simulink model "path_detector"  (Simulink 7.6)
settings: Solver=FixedStepDiscrete  StartTime=0.0  StopTime=0  RelTol=1e-3
values from neighbouring files (symbols this model uses):
  Down_Camera_Dimensions = [120 160]    [VisionConstants.m]
  Iter_Segment_Thresh = 60    [VisionConstants.m]
undefined symbols (not defined in the file or in its folder): a_range, b_range, Rec, SDTV
libraries: vipgeotforms x3, vipconversions x2, viptextngfix x2, viptransforms x2, vipanalysis x1
settings Model: Creator=auvt  LastModifiedBy=auvt  ParamWorkspaceSource=ReferencedWorkspace  TunableVars=Compass_Yaw_Kd,Compass_Yaw_Ki,Compass_Yaw_Kp,Depth_Kd,Depth_Ki,Depth_Kp,Heading_Kd,Heading_Ki,Heading_Kp,IMU_YVel_Kd,IMU_YVel_Ki,IMU_YVel_Kp,IMU_YawRate_Kd,IMU_YawRate_Ki,IMU_YawRate_Kp,Target_Down_X_Kd,Target_Down_X_Ki,Target_Down_X_Kp,Target_Down_Y_Kd,Target_Down_Y_Ki,Target_Down_Y_Kp,Target_Down_Yaw_Kd,Target_Down_Yaw_Ki,Target_Down_Yaw_Kp,Target_Forward_Y_Kd,Target_Forward_Y_Ki,Target_Forward_Y_Kp,Target_Forward_Yaw_Kd,Target_Forward_Yaw_Ki,Target_Forward_Yaw_Kp,Target_Forward_Z_Kd,Target_Forward_Z_Ki,Target_Forward_Z_Kp,Thruster_Friction_Zero,Thruster_LeftAngled_Gain,Thruster_LeftFwd_Gain,Thruster_RightAngled_Gain,Thruster_RightFwd_Gain,ZVelocity_Neg_Max  TunableVarsStorageClass=Auto,Auto,Auto,Auto,Auto,Auto,Auto,Auto,Auto,Auto,Auto,Auto,Auto,Auto,Auto,Auto,Auto,Auto,Auto,Auto,Auto,Auto,Auto,Auto,Auto,Auto,Auto,Auto,Auto,Auto,Auto,Auto,Auto,Auto,Auto,Auto,Auto,Auto,Auto  TunableVarsTypeQualifier=,,,,,,,,,,,,,,,,,,,,,,,,,,,,,,,,,,,,,,
settings MATStruct: SampleTime=0.02  Offset=0  Priority=[1.0]
settings OptimizationCC: InlineParams=on  OptimizeModelRefInitCode=on
settings RTWCC: SystemTargetFile=ert.tlc  GenCodeOnly=on  TemplateMakefile=ert_default_tmf  PostCodeGenCommand=packNGo(buildInfo);  Description=Real-Time Workshop Embedded Coder  GenerateReport=on  ProcessScript=ert_make_rtw_hook  IncludeHyperlinkInReport=on  LaunchReport=on  TargetLang=C++
settings CodeAppCC: IgnoreCustomStorageClasses=off
settings ERTTargetCC: MultiwordLength=2048  GenerateSampleERTMain=on  IncludeMdlTerminateFcn=off  InlinedParameterPlacement=NonHierarchical  ERTCustomFileTemplate=example_file_process.tlc  ConvertIfToSwitch=off

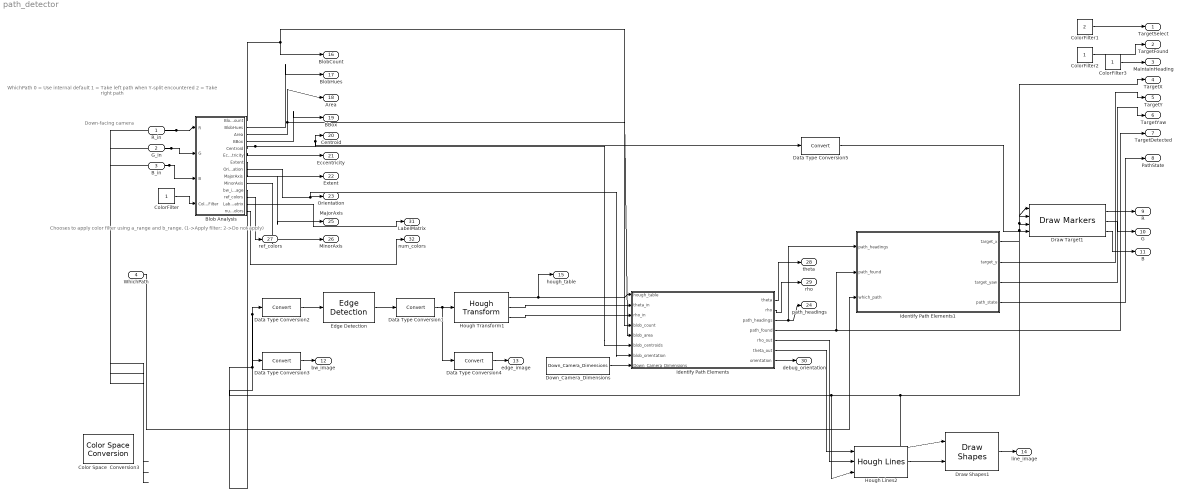
== system path_detector ==
  note: Down-facing camera
  note: WhichPath
      | 0 = Use internal default
      | 1 = Take left path when Y-split encountered
      | 2 = Take right path
  note: Chooses to apply color
      | filter using a_range and
      | b_range. (1->Apply
      | filter; 2->Do not apply)
  R_in : Inport  PortDimensions=Down_Camera_Dimensions
  G_in : Inport  Port=2  PortDimensions=Down_Camera_Dimensions
  B_in : Inport  Port=3  PortDimensions=Down_Camera_Dimensions
  WhichPath : Inport  Port=4
  Blob Analysis : Subsystem
  Color Space  Conversion3 : vipconversions/Color Space  Conversion  conversion=Obsolete  conversionActive=R'G'B' to HSV  wp_str=D50  rec=Rec. 601 (SDTV)  sys=1125/60/2:1  imagePorts=Separate color signals
  ColorFilter : Constant  SampleTime=-1
  ColorFilter1 : Constant  Value=2  SampleTime=-1
  ColorFilter2 : Constant  SampleTime=-1
  ColorFilter3 : Constant  SampleTime=-1
  Data Type Conversion{1..5} (5 alike) : DataTypeConversion
  Down_Camera_Dimensions : Constant  Value=Down_Camera_Dimensions  SampleTime=-1
  Draw Shapes1 : viptextngfix/Draw Shapes  DialogController=vipDDGCreate  DialogControllerArgs=DataTag3  shape=Lines  fill=off  fillClrSource=Specify via dialog  display=User-specified value  intensity=200  color=.2  opacity=0.6  viewport=Entire image  antialiasing=off  inType=Obsolete  imagePorts=One multidimensional signal  prodOutputMode=Binary point scaling  prodOutputWordLength=32  prodOutputFracLength=14  memoryMode=Specify word length  memoryWordLength=16  memoryFracLength=15  roundingMode=Floor  overflowMode=off
  Draw Target1 : viptextngfix/Draw Markers  DialogController=vipDDGCreate  DialogControllerArgs=DataTag4  shape=X-mark  size=7  fill=off  fillClrSource=Specify via dialog  display=Black  intensity=200  color=[0 0 0]  opacity=0.6  viewport=Entire image  antialiasing=off  inType=Obsolete  imagePorts=Separate color signals  prodOutputMode=Binary point scaling  prodOutputWordLength=32  prodOutputFracLength=14  memoryMode=Specify word length  memoryWordLength=16  memoryFracLength=15  roundingMode=Floor  overflowMode=off
  Edge Detection : vipanalysis/Edge Detection  DialogController=vipDDGCreate  DialogControllerArgs=DataTag5  method=Sobel  outputType=Binary image  userDefinedThreshold=off  thresholdSource=Specify via dialog  threshold=20  thresholdTuning=3  edgeThinning=on  threshold_canny=[0.25 0.60]  autoPercent=70  sigma=1  roundingMode=Floor  overflowMode=off
  Hough Lines2 : viptransforms/Hough Lines  DialogController=vipDDGCreate  DialogControllerArgs=DataTag6  sineCompMethod=Trigonometric function  thetaRes=pi/180  firstCoeffMode=Specify word length  firstCoeffWordLength=16  firstCoeffFracLength=15  prodOutputMode=Binary point scaling  prodOutputWordLength=32  prodOutputFracLength=16  roundingMode=Nearest  overflowMode=on
  Hough Transform1 : viptransforms/Hough Transform  DialogController=vipDDGCreate  DialogControllerArgs=DataTag7  theta_res=pi/180  rho_res=1  out_theta_rho=on  outdtmode=double  firstCoeffMode=Binary point scaling  firstCoeffWordLength=16  firstCoeffFracLength=14  secondCoeffMode=Binary point scaling  secondCoeffWordLength=32  secondCoeffFracLength=16  outputMode=Binary point scaling  outputWordLength=16  outputFracLength=0  accumMode=Binary point scaling  accumWordLength=32  accumFracLength=20  prodOutputMode=Binary point scaling  prodOutputWordLength=32  prodOutputFracLength=20  memoryMode=Binary point scaling  memoryWordLength=32  memoryFracLength=16  roundingMode=Nearest  overflowMode=on
  Identify Path Elements : Stateflow chart  TreatAsAtomicUnit=on  SystemSampleTime=[1/30 0]
  Identify Path Elements1 : Stateflow chart  TreatAsAtomicUnit=on  SystemSampleTime=[1/30 0]
  TargetSelect : Outport  OutDataTypeStr=double
  TargetFound : Outport  Port=2  OutDataTypeStr=double
  MaintainHeading : Outport  Port=3  OutDataTypeStr=double
  TargetX : Outport  Port=4  OutDataTypeStr=double
  TargetY : Outport  Port=5  OutDataTypeStr=double
  TargetYaw : Outport  Port=6  OutDataTypeStr=double
  TargetDetected : Outport  Port=7  OutDataTypeStr=double
  PathState : Outport  Port=8  OutDataTypeStr=double
  R : Outport  Port=9  OutDataTypeStr=double
  G : Outport  Port=10  OutDataTypeStr=double
  B : Outport  Port=11  OutDataTypeStr=double
  bw_image : Outport  Port=12  OutDataTypeStr=double
  edge_image : Outport  Port=13  OutDataTypeStr=double
  line_image : Outport  Port=14  OutDataTypeStr=double
  hough_table : Outport  Port=15  OutDataTypeStr=double
  BlobCount : Outport  Port=16
  BlobHues : Outport  Port=17
  Area : Outport  Port=18
  BBox : Outport  Port=19
  Centroid : Outport  Port=20
  Eccentricity : Outport  Port=21
  Extent : Outport  Port=22
  Orientation : Outport  Port=23
  path_headings : Outport  Port=24
  MajorAxis : Outport  Port=25
  MinorAxis : Outport  Port=26
  ref_colors : Outport  Port=27
  theta : Outport  Port=28
  rho : Outport  Port=29
  debug_orientation : Outport  Port=30
  LabelMatrix : Outport  Port=31
  num_colors : Outport  Port=32
  wires:
  Blob Analysis/1(BlobCount) -> BlobCount/1, Identify Path Elements/4(blob_count)
  Blob Analysis/2(BlobHues) -> BlobHues/1
  Blob Analysis/3(Area) -> Area/1, Identify Path Elements/5(blob_area)
  Blob Analysis/4(BBox) -> BBox/1
  Blob Analysis/5(Centroid) -> Centroid/1, Data Type Conversion5/1, Identify Path Elements/6(blob_centroids)
  Blob Analysis/6(Eccentricity) -> Eccentricity/1
  Blob Analysis/7(Extent) -> Extent/1
  Blob Analysis/8(Orientation) -> Orientation/1, Identify Path Elements/7(blob_orientation)
  Blob Analysis/9(MajorAxis) -> MajorAxis/1
  Blob Analysis/10(MinorAxis) -> MinorAxis/1
  Blob Analysis/12(ref_colors) -> ref_colors/1
  R_in/1 -> Blob Analysis/1(R)
  G_in/1 -> Blob Analysis/2(G)
  B_in/1 -> Blob Analysis/3(B)
  Edge Detection/1 -> Data Type Conversion1/1
  Data Type Conversion2/1 -> Edge Detection/1
  Data Type Conversion1/1 -> Hough Transform1/1, Data Type Conversion4/1
  Data Type Conversion3/1 -> bw_image/1
  Data Type Conversion4/1 -> edge_image/1
  Hough Transform1/1 -> Identify Path Elements/1(hough_table), hough_table/1
  Hough Transform1/2 -> Identify Path Elements/2(theta_in)
  Hough Transform1/3 -> Identify Path Elements/3(rho_in)
  Down_Camera_Dimensions/1 -> Identify Path Elements/8(Down_Camera_Dimensions)
  Identify Path Elements/3(path_headings) -> path_headings/1, Identify Path Elements1/1(path_headings)
  Hough Lines2/1 -> Draw Shapes1/2
  Draw Shapes1/1 -> line_image/1
  Draw Target1/1 -> R/1
  Draw Target1/2 -> G/1
  Draw Target1/3 -> B/1
  Data Type Conversion5/1 -> Draw Target1/4
  Identify Path Elements/4(path_found) -> Identify Path Elements1/2(path_found), TargetDetected/1
  Identify Path Elements/1(theta) -> theta/1
  Identify Path Elements/2(rho) -> rho/1
  Identify Path Elements/7(orientation) -> debug_orientation/1
  Identify Path Elements/5(rho_out) -> Hough Lines2/2
  Identify Path Elements/6(theta_out) -> Hough Lines2/1
  Blob Analysis/11(bw_image) -> Data Type Conversion2/1, Data Type Conversion3/1, Hough Lines2/3, Draw Shapes1/1, Draw Target1/1, Draw Target1/2, Draw Target1/3
  WhichPath/1 -> Identify Path Elements1/3(which_path)
  Identify Path Elements1/1(target_x) -> TargetX/1
  Identify Path Elements1/2(target_y) -> TargetY/1
  Identify Path Elements1/3(target_yaw) -> TargetYaw/1
  Identify Path Elements1/4(path_state) -> PathState/1
  ColorFilter/1 -> Blob Analysis/4(ColorFilter)
  ColorFilter1/1 -> TargetSelect/1
  ColorFilter2/1 -> TargetFound/1
  ColorFilter3/1 -> MaintainHeading/1
  Blob Analysis/13(LabelMatrix) -> LabelMatrix/1
  Blob Analysis/14(num_colors) -> num_colors/1

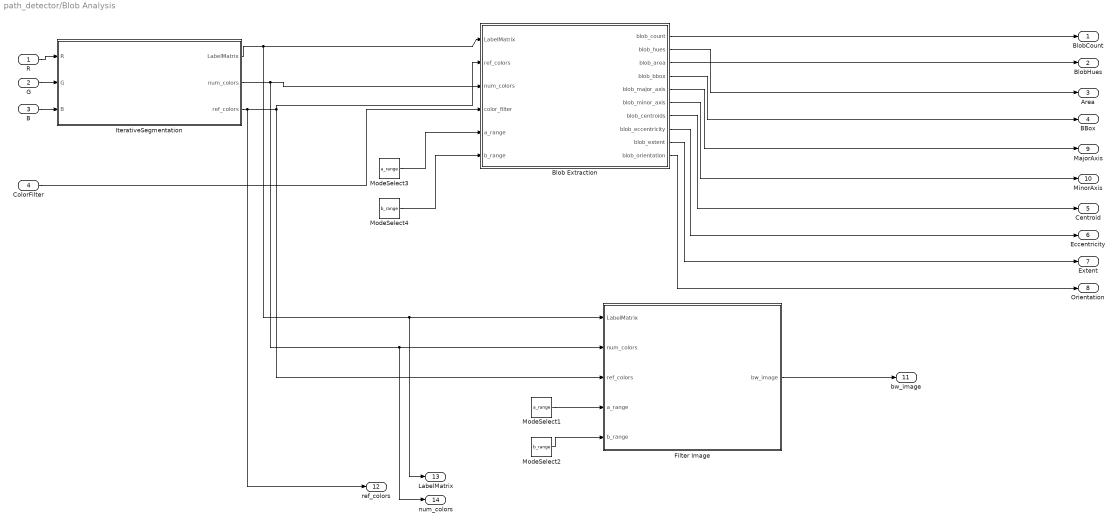
== system path_detector/Blob Analysis ==
  R : Inport
  G : Inport  Port=2
  B : Inport  Port=3
  ColorFilter : Inport  Port=4
  Blob Extraction : Stateflow chart  TreatAsAtomicUnit=on
  Filter Image : Stateflow chart  TreatAsAtomicUnit=on
  IterativeSegmentation : Subsystem
      settings: UndoDeleteFcn=Stateflow.SLINSF.SimulinkMan.restorePreDeleteFcn  PreDeleteFcn=Stateflow.SLINSF.SimulinkMan.removePreDeleteFcn
  ModeSelect1 : Constant  Value=a_range  SampleTime=-1
  ModeSelect2 : Constant  Value=b_range  SampleTime=-1
  ModeSelect3 : Constant  Value=a_range  SampleTime=-1
  ModeSelect4 : Constant  Value=b_range  SampleTime=-1
  BlobCount : Outport
  BlobHues : Outport  Port=2
  Area : Outport  Port=3
  BBox : Outport  Port=4
  Centroid : Outport  Port=5
  Eccentricity : Outport  Port=6
  Extent : Outport  Port=7
  Orientation : Outport  Port=8
  MajorAxis : Outport  Port=9
  MinorAxis : Outport  Port=10
  bw_image : Outport  Port=11
  ref_colors : Outport  Port=12
  LabelMatrix : Outport  Port=13
  num_colors : Outport  Port=14
  wires:
  R/1 -> IterativeSegmentation/1(R)
  G/1 -> IterativeSegmentation/2(G)
  B/1 -> IterativeSegmentation/3(B)
  IterativeSegmentation/1(LabelMatrix) -> Blob Extraction/1(LabelMatrix), Filter Image/1(LabelMatrix), LabelMatrix/1
  IterativeSegmentation/2(num_colors) -> Blob Extraction/3(num_colors), Filter Image/2(num_colors), num_colors/1
  IterativeSegmentation/3(ref_colors) -> Blob Extraction/2(ref_colors), Filter Image/3(ref_colors), ref_colors/1
  Blob Extraction/1(blob_count) -> BlobCount/1
  Blob Extraction/2(blob_hues) -> BlobHues/1
  Blob Extraction/3(blob_area) -> Area/1
  Blob Extraction/4(blob_bbox) -> BBox/1
  Blob Extraction/7(blob_centroids) -> Centroid/1
  Blob Extraction/8(blob_eccentricity) -> Eccentricity/1
  Blob Extraction/9(blob_extent) -> Extent/1
  Blob Extraction/10(blob_orientation) -> Orientation/1
  Blob Extraction/5(blob_major_axis) -> MajorAxis/1
  Blob Extraction/6(blob_minor_axis) -> MinorAxis/1
  ModeSelect1/1 -> Filter Image/4(a_range)
  ModeSelect2/1 -> Filter Image/5(b_range)
  Filter Image/1(bw_image) -> bw_image/1
  ModeSelect3/1 -> Blob Extraction/5(a_range)
  ModeSelect4/1 -> Blob Extraction/6(b_range)
  ColorFilter/1 -> Blob Extraction/4(color_filter)

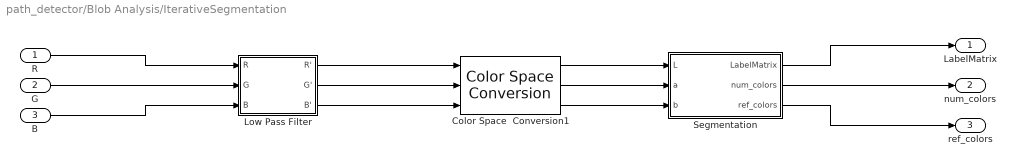
== system path_detector/Blob Analysis/IterativeSegmentation ==
  R : Inport
  G : Inport  Port=2
  B : Inport  Port=3
  Color Space  Conversion1 : vipconversions/Color Space  Conversion  conversion=Obsolete  conversionActive=sR'G'B' to L*a*b*  wp_str=D50  rec=Rec. 601 (SDTV)  sys=1125/60/2:1  imagePorts=Separate color signals
  Low Pass Filter : Subsystem
  Segmentation : Subsystem
  LabelMatrix : Outport
  num_colors : Outport  Port=2
  ref_colors : Outport  Port=3
  wires:
  Segmentation/3(ref_colors) -> ref_colors/1
  Segmentation/2(num_colors) -> num_colors/1
  Segmentation/1(LabelMatrix) -> LabelMatrix/1
  Low Pass Filter/3(B') -> Color Space  Conversion1/3
  Low Pass Filter/2(G') -> Color Space  Conversion1/2
  Low Pass Filter/1(R') -> Color Space  Conversion1/1
  Color Space  Conversion1/3 -> Segmentation/3(b)
  Color Space  Conversion1/2 -> Segmentation/2(a)
  Color Space  Conversion1/1 -> Segmentation/1(L)
  R/1 -> Low Pass Filter/1(R)
  G/1 -> Low Pass Filter/2(G)
  B/1 -> Low Pass Filter/3(B)

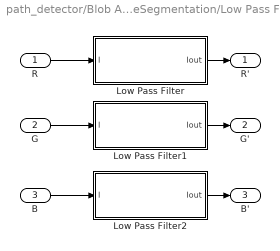
== system path_detector/Blob Analysis/IterativeSegmentation/Low Pass Filter ==
  R : Inport
  G : Inport  Port=2
  B : Inport  Port=3
  Low Pass Filter : Stateflow chart  TreatAsAtomicUnit=on
  Low Pass Filter1 : Stateflow chart  TreatAsAtomicUnit=on
  Low Pass Filter2 : Stateflow chart  TreatAsAtomicUnit=on
  R' : Outport
  G' : Outport  Port=2
  B' : Outport  Port=3
  wires:
  Low Pass Filter/1(Iout) -> R'/1
  Low Pass Filter2/1(Iout) -> B'/1
  Low Pass Filter1/1(Iout) -> G'/1
  B/1 -> Low Pass Filter2/1(I)
  G/1 -> Low Pass Filter1/1(I)
  R/1 -> Low Pass Filter/1(I)

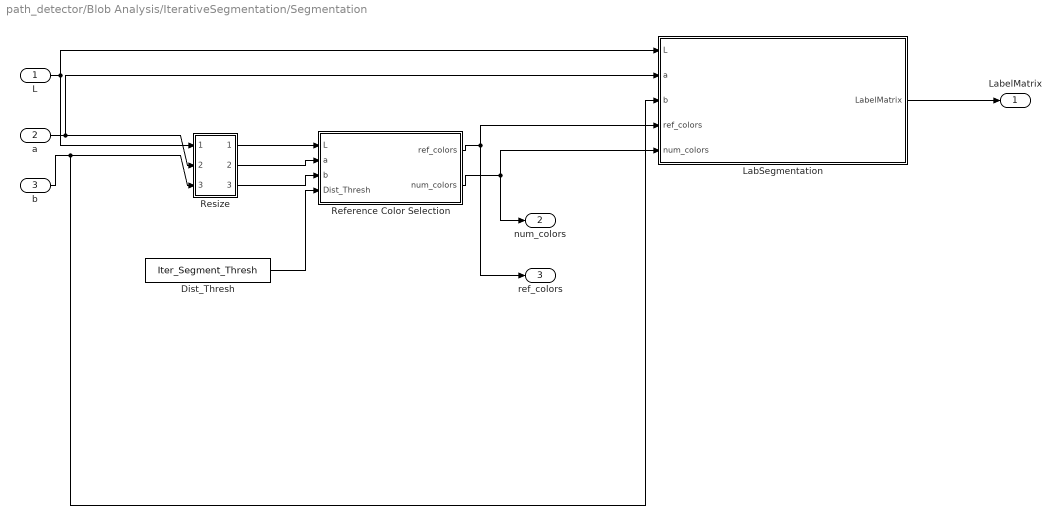
== system path_detector/Blob Analysis/IterativeSegmentation/Segmentation ==
  L : Inport
  a : Inport  Port=2
  b : Inport  Port=3
  Dist_Thresh : Constant  Value=Iter_Segment_Thresh  SampleTime=-1
  LabSegmentation : Stateflow chart  TreatAsAtomicUnit=on
  Reference Color Selection : Stateflow chart  TreatAsAtomicUnit=on
  Resize : Subsystem
  LabelMatrix : Outport
  num_colors : Outport  Port=2
  ref_colors : Outport  Port=3
  wires:
  Dist_Thresh/1 -> Reference Color Selection/4(Dist_Thresh)
  LabSegmentation/1(LabelMatrix) -> LabelMatrix/1
  Reference Color Selection/2(num_colors) -> LabSegmentation/5(num_colors), num_colors/1
  Reference Color Selection/1(ref_colors) -> ref_colors/1, LabSegmentation/4(ref_colors)
  Resize/3(Out3) -> Reference Color Selection/3(b)
  Resize/2(Out2) -> Reference Color Selection/2(a)
  Resize/1(Out1) -> Reference Color Selection/1(L)
  b/1 -> LabSegmentation/3(b), Resize/3(In3)
  a/1 -> LabSegmentation/2(a), Resize/2(In2)
  L/1 -> LabSegmentation/1(L), Resize/1(In1)

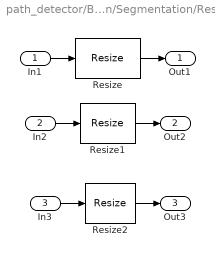
== system path_detector/Blob Analysis/IterativeSegmentation/Segmentation/Resize ==
  In1 : Inport
  In2 : Inport  Port=2
  In3 : Inport  Port=3
  Resize : vipgeotforms/Resize  DialogController=vipDDGCreate  DialogControllerArgs=DataTag0  specify=Number of output rows and columns  rfactor=[]  outCols=25  outRows=25  outRowsCols=[60 80]  interp_method=Bilinear  antialias=on  useROI=off  roiFlag=off  prodOutputMode=Binary point scaling  prodOutputWordLength=32  prodOutputFracLength=10  roundingMode=Nearest  overflowMode=on
  Resize1 : vipgeotforms/Resize  DialogController=vipDDGCreate  DialogControllerArgs=DataTag1  specify=Number of output rows and columns  rfactor=[200 150]  outCols=25  outRows=25  outRowsCols=[60 80]  interp_method=Bilinear  antialias=on  useROI=off  roiFlag=off  prodOutputMode=Binary point scaling  prodOutputWordLength=32  prodOutputFracLength=10  roundingMode=Nearest  overflowMode=on
  Resize2 : vipgeotforms/Resize  DialogController=vipDDGCreate  DialogControllerArgs=DataTag2  specify=Number of output rows and columns  rfactor=[200 150]  outCols=25  outRows=25  outRowsCols=[60 80]  interp_method=Bilinear  antialias=on  useROI=off  roiFlag=off  prodOutputMode=Binary point scaling  prodOutputWordLength=32  prodOutputFracLength=10  roundingMode=Nearest  overflowMode=on
  Out1 : Outport
  Out2 : Outport  Port=2
  Out3 : Outport  Port=3
  wires:
  Resize2/1 -> Out3/1
  In3/1 -> Resize2/1
  Resize1/1 -> Out2/1
  In2/1 -> Resize1/1
  Resize/1 -> Out1/1
  In1/1 -> Resize/1

== matlab function Identify Path Elements1 ==
  data: path_headings input double; path_found input double; target_x output double; target_y output double; target_yaw output double; path_state output double; which_path input double
function [target_x, target_y, target_yaw, path_state] =  choose_path(path_headings, path_found, which_path)
%#eml

% Input
%   which_path = indicates which direction to take; left (1) right (2) or
%     straight (0)

% Return the relative heading of the path element pointing "left" or
%   "right"
if(which_path == 1)
    % Take left path
    target_yaw = min(path_headings)*180/pi;
elseif(which_path == 2)
    % Take right path
    target_yaw = max(path_headings)*180/pi;
else
    % Continue straight
    target_yaw = 0;
end

target_x = 0;
target_y = 0;
path_state = 0;

return

== matlab function Identify Path Elements ==
  data: hough_table input double; theta_in input double; rho_in input double; blob_count input double; blob_area input double; blob_centroids input double; blob_orientation input double; Down_Camera_Dimensions input double; theta output double; rho output double; path_headings output double; path_found output double; rho_out output double; theta_out output double; orientation output double
function [theta, rho, path_headings, path_found, rho_out, theta_out, orientation] = path_detection(hough_table, theta_in, rho_in, blob_count, blob_area, blob_centroids, blob_orientation, Down_Camera_Dimensions)
%#eml

% This function attempts to identfiy path elements, and returns lines,
%   information about the paths that are present, and a true/false
%   path_found parameter.
%
% 5-30-11
%
% Input
%
% Output
%  path_headings = vector of path orientations in terms of headings
%    relative to the auv (degrees)
%  rho, theta = vectors containing lines determined by Hough Transform,
%    ordered by number of votes
%
% Notes:
%   The hough_table is destroyed in this function (acceptable if
%     hough_table is not an output)
%   blob_orientation is destroyed


% Initialize
max_num_lines = 200;  % Considers this many popular lines as candidates
max_num_paths = 3;

[rho_length, theta_length] = size(hough_table);
rows = Down_Camera_Dimensions(1);
cols = Down_Camera_Dimensions(2);
image_area = rows*cols;

rho_tol = .1*max(rows,cols);  % Tolerance within which two lines are coincident
theta_tol = 10*pi/180;  % Tolerence within which two slopes are equal (radians)
area_thresh = 0.8;  % Ratio of blob area to image area considered to imply the blob is actually background noise

rho = zeros(1,max_num_lines);
theta = zeros(1,max_num_lines);
theta_hold = zeros(1,max_num_lines);  % theta_hold is a copy of theta which gets destroyed

rho_out = zeros(1,max_num_lines);
theta_out = zeros(1,max_num_lines);

path_headings = zeros(1,max_num_paths);
path_locations = zeros(2,max_num_paths);
path_found = 0;

% Identify the most likely max_num_lines lines
for( m = 1:max_num_lines )
    
    max_votes = 0;
    i_index = 1;
    j_index = 1;
    for i = 1:rho_length
        for j = 1:theta_length
            if( hough_table(i,j) > max_votes )
                i_index = i;
                j_index = j;
                max_votes = hough_table(i,j);
            end
        end
    end
    
    if(max_votes == 0)
        break;
    end
    
    rho(m) = rho_in(i_index);
    theta(m) = theta_in(j_index);
    theta_hold(m) = theta_in(j_index);
    hough_table(i_index,j_index) = 0;
    
end    


% Correct orientations to vehicle coordinates
for j = 1:blob_count
    % theta_hold:
    %   -is between [-pi/2, +pi/2]
    % blob_orientation:
    %   -is potentially outside this range
    %   -needs to be corrected by pi/2 to get relative heading
%    blob_orientation(j) = (pi/2) - blob_orientation(j);

    blob_orientation(j) = mod(pi - blob_orientation(j), pi) - pi/2;
%    if(blob_orientation(j) > pi/2)
%        blob_orientation(j) = blob_orientation(j) - pi;
%    elseif(blob_orientation(j) < -pi/2)
%        blob_orientation(j) = blob_orientation(j) + pi;
%    end
end


% Compare most popular lines with blob orientations
c = 1;
for p = 1:max_num_paths
    
    found = 0;
    for i = 1:max_num_lines
        for j = 1:blob_count
            
            % Search for a match between one blob and one line
            if( abs(theta_hold(i) - blob_orientation(j)) <= theta_tol  &&  blob_area(j)/image_area <= area_thresh  &&  (theta_hold(i) ~= 1000 && blob_orientation(j) ~= 1000) )
                path_headings(p) = theta_hold(i);
                path_locations(1,p) = blob_centroids(1,j);
                path_locations(2,p) = blob_centroids(2,j);
                
                
                
                %
                rho_out(c) = rho(i);
                theta_out(c) = theta(i);
                c = c + 1;
                %/
                
                
                theta_hold(i) = 1000;  % Invalid angle; do not want this line to be selected again
                blob_orientation(j) = 1000;
                found = 1;
                break;
            end
            
        end
        
        if(found == 1)
            break;
        end
    end
    
end


% Order path_headings to reflect actual path locations (left to right in
%   image)
value = Down_Camera_Dimensions(2).*ones(1,max_num_paths);
j_index = ones(1,max_num_paths);
found = zeros(1,max_num_paths);

for p = 1:max_num_paths
    for j = 1:max_num_paths
        if(path_locations(2,j) < value(p) && found(j) == 0)
            value(p) = path_locations(2,j);
            j_index(p) = j;
        end
    end
    found(j_index(p)) = 1;
end

matr = [path_headings; path_locations];
for p = 1:max_num_paths
    path_headings(p) = matr(1,j_index(p));
    path_locations(1,p) = matr(2,j_index(p));
    path_locations(2,p) = matr(3,j_index(p));
end


















% old code \/ \/

% Determine which way the 'Y' shape is pointing
%path_headings = sort(path_headings, 2, 'ascend');
%heading_diff = abs([ path_headings(2) - path_headings(1), path_headings(3) - path_headings(2), path_headings(1) - path_headings(3)]);
%if(heading_diff(1) < heading_diff(2) && heading_diff(1) < heading_diff(3))
%    y_heading = path_headings(3);
%elseif(heading_diff(2) < heading_diff(1) && heading_diff(2) < heading_diff(3))
%    y_heading = path_headings(1);
%elseif(heading_diff(3) < heading_diff(1) && heading_diff(3) < heading_diff(2))
%    y_heading = path_headings(2);
%else
%    y_heading = 0;
%end




% Determine a good approximation of the median lines (ignore effectively
%   duplicate lines)
%{
rho(1) = rho(1);
theta(1) = theta(1);

m = 2;
for i = 2:max_num_lines
    
    % If rho, theta do not match within tolerance, then store as the next
    %   line
    if( abs(rho(i) - rho(i-1)) >= 30 )
        rho_out(m) = rho(i);
        theta_out(m) = theta(i);
        m = m + 1;
        if( m > 3 )
            break;
        end
    end
    
end




% Select the most popular lines assuming that they correspond to the path
%   edges
%}




theta = theta_hold;
orientation = blob_orientation;

return

== matlab function Blob Analysis/Blob Extraction ==
  data: LabelMatrix input double; ref_colors input double; num_colors input double; color_filter input double; blob_count output double; blob_hues output double; blob_area output double; blob_bbox output double; blob_major_axis output double; blob_minor_axis output double; blob_centroids output double; blob_eccentricity output double; blob_extent output double; blob_orientation output double; a_range input double; b_range input double
function [blob_count, blob_hues, blob_area, blob_bbox, blob_major_axis, blob_minor_axis, blob_centroids, blob_eccentricity, blob_extent, blob_orientation] = GetBlobInfo(LabelMatrix, ref_colors, num_colors, color_filter, a_range, b_range)

% This function extracts 
% Input
%   

% Initialize
max_num_blobs = 50;
min_blob_area = 5;

[rows, cols] = size(LabelMatrix);
LogicMatrix = false(rows,cols);

blob_count = 0;
blob_hues = zeros(3,max_num_blobs);

blob_area = -1.*ones(1,max_num_blobs);
blob_bbox = zeros(4,max_num_blobs);
blob_major_axis = zeros(1,max_num_blobs);
blob_minor_axis = zeros(1,max_num_blobs);
blob_centroids = zeros(2,max_num_blobs);
blob_eccentricity = zeros(1,max_num_blobs);
blob_extent = zeros(1,max_num_blobs);
blob_orientation = zeros(1,max_num_blobs);


% Input hblob, a matrix containing [Area, blob_centroids, Eccentricity] for each
% identified blob
persistent hblob
if isempty(hblob)
    hblob = video.BlobAnalysis('AreaOutputPort',true,'CentroidOutputPort',true,...
        'BoundingBoxOutputPort',true,'MajorAxisLengthOutputPort',true,'MinorAxisLengthOutputPort',true,...
        'OrientationOutputPort',true,...
        'EccentricityOutputPort',true,'ExtentOutputPort',true,'NumBlobsOutputPort',true,...
        'MinimumBlobAreaSource','Property','MinimumBlobArea', min_blob_area);
end


% Calculate geometric information about the blobs
%
% LogicMatrix is a binary version of LabelMatrix, with ones at all
%   locations for which color values are k, and zeros everywhere else
for k = 1:num_colors

    a = ref_colors(k, 2);
    b = ref_colors(k, 3);

    if( color_filter == 1 && a >= a_range(1,5) && a <= a_range(2,5) && b >= b_range(1,5) && b <= b_range(2,5) )

        for i = 1:rows
            for j = 1:cols
                if(LabelMatrix(i,j) ~= k)
                    LogicMatrix(i,j) = false;
                else
                    LogicMatrix(i,j) = true;
                end
            end
        end

        [TArea,TCentroid,TBBox,TMajorAxis,TMinorAxis,TOrientation,TEccent,TExtent,TNumBlobs] = step(hblob,LogicMatrix);

        for i = 1:TNumBlobs
            if(blob_count + TNumBlobs <= max_num_blobs)

                blob_centroids(1,blob_count+i) = TCentroid(1,i);
                blob_centroids(2,blob_count+i) = TCentroid(2,i);

                ii = round(blob_centroids(1,blob_count+i));
                jj = round(blob_centroids(2,blob_count+i));

                blob_hues(1,blob_count+i) = ref_colors( LabelMatrix(ii,jj), 1 );
                blob_hues(2,blob_count+i) = ref_colors( LabelMatrix(ii,jj), 2 );
                blob_hues(3,blob_count+i) = ref_colors( LabelMatrix(ii,jj), 3 );

                blob_area(blob_count+i) = TArea(i);
                blob_bbox(blob_count+i) = TBBox(i);
                blob_major_axis(blob_count+i) = TMajorAxis(i);
                blob_minor_axis(blob_count+i) = TMinorAxis(i);
                blob_eccentricity(blob_count+i) = TEccent(i);
                blob_extent(blob_count+i) = TExtent(i);
                blob_orientation(blob_count+i) = TOrientation(i);

            end
        end

        blob_count = blob_count + double(TNumBlobs);

    end
    
end


return

== matlab function Blob Analysis/Filter Image ==
  data: LabelMatrix input double; num_colors input double; ref_colors input double; bw_image output double; a_range input double; b_range input double
function bw_image = Filter_Image(LabelMatrix, num_colors, ref_colors, a_range, b_range)


% Initialize
[rows,cols] = size(LabelMatrix);
bw_image = zeros(rows,cols);


% Allow only colors in specified range
for r = 1:rows
    for c = 1:cols
        
        a = ref_colors(LabelMatrix(r,c), 2);
        b = ref_colors(LabelMatrix(r,c), 3);
        
        if( a >= a_range(1,5) && a <= a_range(2,5) && b >= b_range(1,5) && b <= b_range(2,5) )
            bw_image(r,c) = 1;
        end
        
    end
end


return

== matlab function Blob Analysis/IterativeSegmentation/Low Pass Filter/Low Pass Filter ==
  data: I input double; Iout output double
function Iout = GaussianBlurr(I)
% This function calculates the gaussian blur of an intensity image

sigma = sqrt(2);

Grows = 3;    % Gaussian matrix rows
Gcols = 3;    % Gaussian matrix columns

[Irows Icols] = size(I);

Iout = double(zeros(Irows,Icols));

Trows = Irows - Grows + 1;
Tcols = Icols - Gcols + 1;
Itemp = double(zeros(Trows,Tcols));

G = zeros(Grows,Gcols);

FirstRow = ceil(-Grows/2);
LastRow = floor(Grows/2);
FirstCol = ceil(-Gcols/2);
LastCol = floor(Gcols/2);
Gsum = 0;
for i=FirstRow:LastRow
    for j = FirstCol:LastCol
        G(i-FirstRow+1,j-FirstCol+1) = exp(-(j*j+i*i)/(2*sigma*sigma));
        Gsum = Gsum + G(i-FirstRow+1,j-FirstCol+1);
    end
end

G = G./Gsum;

Itemp = conv2(double(I),double(G),'valid');

% reflect boundaries to keep image the same size
% top
Iout((1:LastRow),(LastCol+1:Icols-LastCol)) = Itemp((1:LastRow),(1:Tcols));
% bottom
Iout((Irows-LastRow+1:Irows),(LastCol+1:Icols-LastCol)) = Itemp((Trows-LastRow+1:Trows),(1:Tcols));
% left
Iout((1+LastRow:Irows-LastRow),(1:LastCol)) = Itemp((1:Trows),(1:LastCol));
% right
Iout((1+LastRow:Irows-LastRow),(Icols-LastCol+1:Icols)) = Itemp((1:Trows),(Tcols-LastCol+1:Tcols));
% center
Iout((1+LastRow:Irows-LastRow),(1+LastCol:Icols-LastCol)) = Itemp;
% top left corner
Iout(1:LastRow,1:LastCol) = Itemp(1:LastRow,1:LastCol);
% top right corner
Iout(1:LastRow,Icols-LastCol:Icols) = Itemp(1:LastRow,Tcols-LastCol:Tcols);
% bottom left corner
Iout(Irows-LastRow:Irows,1:LastCol) = Itemp(Trows-LastRow:Trows,1:LastCol);
% bottom right corner
Iout(Irows-LastRow:Irows,Icols-LastCol:Icols) = Itemp(Trows-LastRow:Trows,Tcols-LastCol:Tcols);

return

== matlab function Blob Analysis/IterativeSegmentation/Low Pass Filter/Low Pass Filter1 ==
  data: I input double; Iout output double
function Iout = GaussianBlurr(I)
% This function calculates the gaussian blur of an intensity image

sigma = sqrt(2);

Grows = 3;    % Gaussian matrix rows
Gcols = 3;    % Gaussian matrix columns

[Irows Icols] = size(I);

Iout = double(zeros(Irows,Icols));

Trows = Irows - Grows + 1;
Tcols = Icols - Gcols + 1;
Itemp = double(zeros(Trows,Tcols));

G = zeros(Grows,Gcols);

FirstRow = ceil(-Grows/2);
LastRow = floor(Grows/2);
FirstCol = ceil(-Gcols/2);
LastCol = floor(Gcols/2);
Gsum = 0;
for i=FirstRow:LastRow
    for j = FirstCol:LastCol
        G(i-FirstRow+1,j-FirstCol+1) = exp(-(j*j+i*i)/(2*sigma*sigma));
        Gsum = Gsum + G(i-FirstRow+1,j-FirstCol+1);
    end
end

G = G./Gsum;

Itemp = conv2(double(I),double(G),'valid');

% reflect boundaries to keep image the same size
% top
Iout((1:LastRow),(LastCol+1:Icols-LastCol)) = Itemp((1:LastRow),(1:Tcols));
% bottom
Iout((Irows-LastRow+1:Irows),(LastCol+1:Icols-LastCol)) = Itemp((Trows-LastRow+1:Trows),(1:Tcols));
% left
Iout((1+LastRow:Irows-LastRow),(1:LastCol)) = Itemp((1:Trows),(1:LastCol));
% right
Iout((1+LastRow:Irows-LastRow),(Icols-LastCol+1:Icols)) = Itemp((1:Trows),(Tcols-LastCol+1:Tcols));
% center
Iout((1+LastRow:Irows-LastRow),(1+LastCol:Icols-LastCol)) = Itemp;
% top left corner
Iout(1:LastRow,1:LastCol) = Itemp(1:LastRow,1:LastCol);
% top right corner
Iout(1:LastRow,Icols-LastCol:Icols) = Itemp(1:LastRow,Tcols-LastCol:Tcols);
% bottom left corner
Iout(Irows-LastRow:Irows,1:LastCol) = Itemp(Trows-LastRow:Trows,1:LastCol);
% bottom right corner
Iout(Irows-LastRow:Irows,Icols-LastCol:Icols) = Itemp(Trows-LastRow:Trows,Tcols-LastCol:Tcols);

return

== matlab function Blob Analysis/IterativeSegmentation/Low Pass Filter/Low Pass Filter2 ==
  data: I input double; Iout output double
function Iout = GaussianBlurr(I)
% This function calculates the gaussian blur of an intensity image

sigma = sqrt(2);

Grows = 3;    % Gaussian matrix rows
Gcols = 3;    % Gaussian matrix columns

[Irows Icols] = size(I);

Iout = double(zeros(Irows,Icols));

Trows = Irows - Grows + 1;
Tcols = Icols - Gcols + 1;
Itemp = double(zeros(Trows,Tcols));

G = zeros(Grows,Gcols);

FirstRow = ceil(-Grows/2);
LastRow = floor(Grows/2);
FirstCol = ceil(-Gcols/2);
LastCol = floor(Gcols/2);
Gsum = 0;
for i=FirstRow:LastRow
    for j = FirstCol:LastCol
        G(i-FirstRow+1,j-FirstCol+1) = exp(-(j*j+i*i)/(2*sigma*sigma));
        Gsum = Gsum + G(i-FirstRow+1,j-FirstCol+1);
    end
end

G = G./Gsum;

Itemp = conv2(double(I),double(G),'valid');

% reflect boundaries to keep image the same size
% top
Iout((1:LastRow),(LastCol+1:Icols-LastCol)) = Itemp((1:LastRow),(1:Tcols));
% bottom
Iout((Irows-LastRow+1:Irows),(LastCol+1:Icols-LastCol)) = Itemp((Trows-LastRow+1:Trows),(1:Tcols));
% left
Iout((1+LastRow:Irows-LastRow),(1:LastCol)) = Itemp((1:Trows),(1:LastCol));
% right
Iout((1+LastRow:Irows-LastRow),(Icols-LastCol+1:Icols)) = Itemp((1:Trows),(Tcols-LastCol+1:Tcols));
% center
Iout((1+LastRow:Irows-LastRow),(1+LastCol:Icols-LastCol)) = Itemp;
% top left corner
Iout(1:LastRow,1:LastCol) = Itemp(1:LastRow,1:LastCol);
% top right corner
Iout(1:LastRow,Icols-LastCol:Icols) = Itemp(1:LastRow,Tcols-LastCol:Tcols);
% bottom left corner
Iout(Irows-LastRow:Irows,1:LastCol) = Itemp(Trows-LastRow:Trows,1:LastCol);
% bottom right corner
Iout(Irows-LastRow:Irows,Icols-LastCol:Icols) = Itemp(Trows-LastRow:Trows,Tcols-LastCol:Tcols);

return

== matlab function Blob Analysis/IterativeSegmentation/Segmentation/LabSegmentation ==
  data: L input double; LabelMatrix output double; a input double; b input double; ref_colors input double; num_colors input double
function LabelMatrix  = LabSegmentation(L,a,b,ref_colors,num_colors)
% This function generates the label matrix

[rows cols] = size(L);

Lout = zeros(rows,cols);
aout = zeros(rows,cols);
bout = zeros(rows,cols);

LabelMatrix = zeros(rows,cols);

for i = 1:rows
    for j = 1:cols
        min_dist = 1000;
        index = 1;
        for k = 1:num_colors
            dist = sqrt((ref_colors(k,1) - L(i,j))^2 + (ref_colors(k,2) - a(i,j))^2 + (ref_colors(k,3) - b(i,j))^2);
            if(dist < min_dist)
                min_dist = double(dist);
                index = k;
            end
        end
        LabelMatrix(i,j) = index;
    end
end

for i = 1:rows
    for j = 1:cols
        Lout(i,j) = ref_colors(LabelMatrix(i,j),1);
        aout(i,j) = ref_colors(LabelMatrix(i,j),2);
        bout(i,j) = ref_colors(LabelMatrix(i,j),3);
    end
end

cow = 1;

return

== matlab function Blob Analysis/IterativeSegmentation/Segmentation/Reference Color Selection ==
  data: L input double; ref_colors output double; a input double; b input double; num_colors output double; Dist_Thresh input double
function [ref_colors, num_colors] = Segmentation(L,a,b,Dist_Thresh)
% This function tries segmentation by adding new reference colors everytime
% a pixel is found with a distance greater than a certain amount from
% every other reference color

[rows cols] = size(L);

Dist_Threshold = Dist_Thresh;% L = 0 to 100, a = -100 to 100, b = -100 to 100
                    % max dist = 300 -> 60/300 is 20%
x = 1;  % coefficients determining distance calculation
y = 1.5;
z = 1.5;

max_num_colors = 50;
ref_colors = zeros(max_num_colors,3);   % At most 50 different reference colors
LabelMatrix = zeros(rows,cols);
num_colors = 1;

center_row = floor(rows/2);
center_col = floor(cols/2);

% Define first reference color to be colr
ref_colors(1,:) = [L(center_row,center_col) a(center_row,center_col) b(center_row,center_col)];

flag = 0;
i = 1;
j = 1;
while(i <= rows)        % perform initial segmentation
    while(i <= rows && flag == 0)
        while(j <= cols && flag == 0)
            k = 1;
            min_dist = 1000;
            index = 1;
            while(k <= num_colors)
                dist = sqrt(x*(ref_colors(k,1) - L(i,j))^2 + y*(ref_colors(k,2) - a(i,j))^2 + z*(ref_colors(k,3) - b(i,j))^2);
                if(min_dist > dist)
                    min_dist = double(dist);
                    index = k;
                end
                k = k + 1;
            end
            if(j == 117)
                cow = 1;
            end
            if(min_dist > Dist_Threshold && num_colors < max_num_colors)
                ref_colors(num_colors+1,:) = [L(i,j) a(i,j) b(i,j)];
                num_colors = num_colors + 1;
                flag = 1;
                i = 0;
                j = 0;
            else
                LabelMatrix(i,j) = index;
            end
            j = j + 1;
        end
        j = 1;
        i = i + 1;
    end
    flag = 0;
end

% Go through image once more to get more accurate values for the different regions
ref_color_L_avg = zeros(50,1);
ref_color_a_avg = zeros(50,1);
ref_color_b_avg = zeros(50,1);
color_count = zeros(50,1);
for i = 1:rows
    for j = 1:cols
        index = LabelMatrix(i,j);
        ref_color_L_avg(index) = ref_color_L_avg(index) + L(i,j);
        ref_color_a_avg(index) = ref_color_a_avg(index) + a(i,j);
        ref_color_b_avg(index) = ref_color_b_avg(index) + b(i,j);
        color_count(index) = color_count(index) + 1;
    end
end
ref_color_L_avg = ref_color_L_avg ./ color_count;
ref_color_a_avg = ref_color_a_avg ./ color_count;
ref_color_b_avg = ref_color_b_avg ./ color_count;

for i = 1:num_colors
    ref_colors(i,1) = ref_color_L_avg(i);
    ref_colors(i,2) = ref_color_a_avg(i);
    ref_colors(i,3) = ref_color_b_avg(i);
end

return
